simulink model "receiver"  (R2021b)
settings: Solver=VariableStepAuto  StartTime=0.0  StopTime=10000/3.2e6  RelTol=1e-3
PreLoadFcn:
  | setup_receiver
InitFcn:
  | setup_receiver
values from neighbouring files (symbols this model uses):
  fir_bbuf = reshape([fir_barker_13; fir_barker_13; fir_barker_13], [1, length(fir_barker_13)*3])    [setup_receiver.m]
  tx_data = [tx_data mbuf]    [setup_receiver.m]
undefined symbols (not defined in the file or in its folder): AXI4, designMultirateFIR, Lite, xlfda_numerator
libraries: hdlBasic x467, hdlsllib x15, dspmlti4 x8, hdlDSPIP x6, hdlSSR x6, dspswit3 x4, hdlUtilities x3, commrandsrc3 x2, dspsigops x2, simulink x1, vmcUtilities x1
(part 2 of 6)

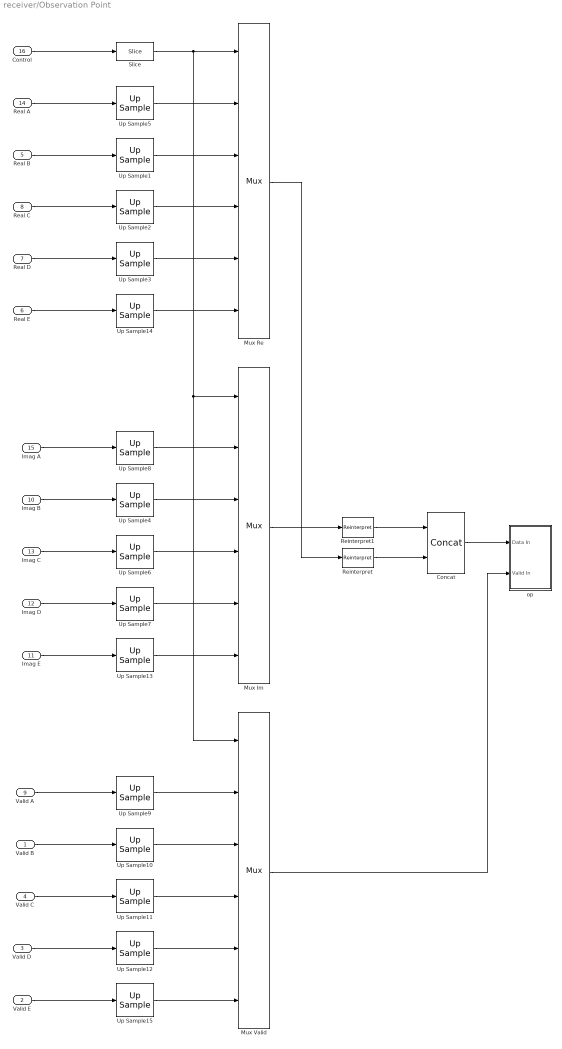
== system receiver/Observation Point ==
  Valid B : Inport
  Valid E : Inport  Port=2
  Valid D : Inport  Port=3
  Valid C : Inport  Port=4
  Real B : Inport  Port=5
  Real E : Inport  Port=6
  Real D : Inport  Port=7
  Real C : Inport  Port=8
  Valid A : Inport  Port=9
  Imag B : Inport  Port=10
  Imag E : Inport  Port=11
  Imag D : Inport  Port=12
  Imag C : Inport  Port=13
  Real A : Inport  Port=14
  Imag A : Inport  Port=15
  Control : Inport  Port=16
  Concat : hdlBasic/Concat  num_inputs=2  XmcBlockStatus=1  maskContainerNames=group1  block_type=concat  block_config=sysgen:Concat_config
  Mux Im : hdlBasic/Mux  inputs=5  en=off  latency=1  precision=Full  arith_type=Unsigned  n_bits=16  bin_pt=14  quantization=Truncate  overflow=Wrap  XmcBlockStatus=1  maskContainerNames=tabcontainer1  block_type=mux  block_config=sysgen:Mux_config
  Mux Re : hdlBasic/Mux  inputs=5  en=off  latency=1  precision=Full  arith_type=Unsigned  n_bits=16  bin_pt=14  quantization=Truncate  overflow=Wrap  XmcBlockStatus=1  maskContainerNames=tabcontainer1  block_type=mux  block_config=sysgen:Mux_config
  Mux Valid : hdlBasic/Mux  inputs=5  en=off  latency=1  precision=Full  arith_type=Unsigned  n_bits=16  bin_pt=14  quantization=Truncate  overflow=Wrap  XmcBlockStatus=1  maskContainerNames=tabcontainer1  block_type=mux  block_config=sysgen:Mux_config
  Reinterpret : hdlBasic/Reinterpret  force_arith_type=on  arith_type=Unsigned  force_bin_pt=on  bin_pt=0  XmcBlockStatus=1  maskContainerNames=group1  block_type=reinterpret  block_config=sysgen:Reinterpret_config
  Reinterpret1 : hdlBasic/Reinterpret  force_arith_type=on  arith_type=Unsigned  force_bin_pt=on  bin_pt=0  XmcBlockStatus=1  maskContainerNames=group1  block_type=reinterpret  block_config=sysgen:Reinterpret_config
  Slice : hdlBasic/Slice  nbits=1  boolean_output=off  mode=Two Bit Locations  bit1=2  base1=LSB of Input  bit0=0  base0=LSB of Input  XmcBlockStatus=1  maskContainerNames=group1  block_type=slice  block_config=sysgen:Slice_config
  Up Sample{1..2,4..6,8} (6 alike) : hdlBasic/Up Sample  sample_ratio=64e6/3.2e6  copy_samples=on  en=off  latency=0  XmcBlockStatus=1  maskContainerNames=group1  block_type=usamp  block_config=sysgen:Upsample_config
  Up Sample10 : hdlBasic/Up Sample  sample_ratio=64e6/3.2e6  copy_samples=off  en=off  latency=0  XmcBlockStatus=1  maskContainerNames=group1  block_type=usamp  block_config=sysgen:Upsample_config
  Up Sample11 : hdlBasic/Up Sample  sample_ratio=64e6/3.2e6  copy_samples=off  en=off  latency=0  XmcBlockStatus=1  maskContainerNames=group1  block_type=usamp  block_config=sysgen:Upsample_config
  Up Sample12 : hdlBasic/Up Sample  sample_ratio=64e6/12.8e6  copy_samples=off  en=off  latency=0  XmcBlockStatus=1  maskContainerNames=group1  block_type=usamp  block_config=sysgen:Upsample_config
  Up Sample{3,7,13..14} (4 alike) : hdlBasic/Up Sample  sample_ratio=64e6/12.8e6  copy_samples=on  en=off  latency=0  XmcBlockStatus=1  maskContainerNames=group1  block_type=usamp  block_config=sysgen:Upsample_config
  Up Sample15 : hdlBasic/Up Sample  sample_ratio=64e6/12.8e6  copy_samples=off  en=off  latency=0  XmcBlockStatus=1  maskContainerNames=group1  block_type=usamp  block_config=sysgen:Upsample_config
  Up Sample9 : hdlBasic/Up Sample  sample_ratio=64e6/3.2e6  copy_samples=off  en=off  latency=0  XmcBlockStatus=1  maskContainerNames=group1  block_type=usamp  block_config=sysgen:Upsample_config
  op : Subsystem
  wires:
  Valid B/1 -> Up Sample10/1
  Up Sample10/1 -> Mux Valid/3
  Control/1 -> Slice/1
  Up Sample1/1 -> Mux Re/3
  Concat/1 -> op/1(Data In)
  Mux Re/1 -> Reinterpret/1
  Real B/1 -> Up Sample1/1
  Up Sample11/1 -> Mux Valid/4
  Up Sample2/1 -> Mux Re/4
  Mux Valid/1 -> op/2(Valid In)
  Up Sample3/1 -> Mux Re/5
  Up Sample6/1 -> Mux Im/4
  Up Sample12/1 -> Mux Valid/5
  Imag A/1 -> Up Sample8/1
  Real A/1 -> Up Sample5/1
  Reinterpret/1 -> Concat/2
  Up Sample7/1 -> Mux Im/5
  Reinterpret1/1 -> Concat/1
  Imag C/1 -> Up Sample6/1
  Up Sample5/1 -> Mux Re/2
  Up Sample4/1 -> Mux Im/3
  Up Sample8/1 -> Mux Im/2
  Mux Im/1 -> Reinterpret1/1
  Up Sample9/1 -> Mux Valid/2
  Valid A/1 -> Up Sample9/1
  Imag D/1 -> Up Sample7/1
  Valid D/1 -> Up Sample12/1
  Real D/1 -> Up Sample3/1
  Valid C/1 -> Up Sample11/1
  Valid E/1 -> Up Sample15/1
  Imag E/1 -> Up Sample13/1
  Real C/1 -> Up Sample2/1
  Imag B/1 -> Up Sample4/1
  Real E/1 -> Up Sample14/1
  Slice/1 -> Mux Valid/1, Mux Im/1, Mux Re/1
  Up Sample13/1 -> Mux Im/6
  Up Sample14/1 -> Mux Re/6
  Up Sample15/1 -> Mux Valid/6

== system receiver/QPSK System ==
  Enable : Inport
  Complex to Real-Imag : ComplexToRealImag
  QPSK TX Generation : Subsystem
  RF Balun Gain RX : Gain  Gain=1/2
  RF Balun Gain TX : Gain  Gain=1/2
  RF-ADC : Subsystem  mask{fs_ghz=1.024, decim=8x, ssr=2, mode=Fine, fc=0.064100, fph=0, fcoarse=fs/4}
      mask prompts: fs_ghz "Sample Rate (GHz):"; decim "Interpolation Mode:"; ssr "Samples per AXI4-Stream Cycle:"; mode "Mixer Type:"; fc "NCO Frequency (GHz):"; fph "NCO Phase (Rads):"; fcoarse "Frequency:"
      mask init:
      | % Obtain the sample rate in Hz
      | fs = str2double(get_param(gcb, 'fs_ghz'))*1e9;
      | 
      | % Set the mode of the RF-DAC interpolation filter
      | switch get_param(gcb, 'decim')
      |     case '1x'
      |         D = 1;
      |     case '2x'
      |         D = 2;
      |     case '4x'
      |         D = 4;
      |     case '8x'
      |         D = 8;
      |     otherwise
      |         D = 1;
      | end
      | 
      | % Get the AXI-Stream clock for display to user
      | axi_clk = (fs/(str2double(get_param(gcb, 'ssr'))*D))*1e-6;
      | 
      | % Get the block mask object to manipulate settings
      | mo = get_param(gcb, 'MaskObject');
      | 
      | % Update text to display the required AXI-Stream clock
      | tc = mo.getDialogControl('axi_text');
      | tc.Prompt = ['      Required AXI-Stream Clock: ', num2str(axi_clk), ' MHz'];
      | 
      | % Set the RF-DAC Mixer mode
      | switch get_param(gcb, 'mode')
      |     case 'Bypass'
      |         m = 0;
      |     case 'Coarse'
      |         m = 1;
      |     case 'Fine'
      |         m = 2;
      |     otherwise
      |         m = 0;
      | end
      | 
      | % Set the RF-DAC Coarse Mixer mode
      | switch get_param(gcb, 'fcoarse')
      |     case 'fs/2'
      |         mc = 0;
      |     case 'fs/4'
      |         mc = 1;
      |     case '-fs/4'
      |         mc = 2;
      |     otherwise
      |         mc = 0;
      | end
      | 
      | % Set other blocks
      | set_param([gcb, '/Decimation Filter'], 'decim', get_param(gcb, 'decim'));
      mask Callback fs_ghz:
      | % Obtain the sample rate in Hz
      | fs = str2double(get_param(gcb, 'fs_ghz'))*1e9;
      | 
      | % Set the mode of the RF-DAC interpolation filter
      | switch get_param(gcb, 'decim')
      |     case '1x'
      |         D = 1;
      |     case '2x'
      |         D = 2;
      |     case '4x'
      |         D = 4;
      |     case '8x'
      |         D = 8;
      |     otherwise
      |         D = 1;
      | end
      | 
      | % Get the AXI-Stream clock for display to user
      | axi_clk = (fs/(str2double(get_param(gcb, 'ssr'))*D))*1e-6;
      | 
      | % Get the block mask object to manipulate settings
      | mo = get_param(gcb, 'MaskObject');
      | 
      | % Update text to display the required AXI-Stream clock
      | tc = mo.getDialogControl('axi_text');
      | tc.Prompt = ['      Required AXI-Stream Clock: ', num2str(axi_clk), ' MHz'];
      mask TypeOptions decim: 1x | 2x | 4x | 8x
      mask Callback decim:
      | % Obtain the sample rate in Hz
      | fs = str2double(get_param(gcb, 'fs_ghz'))*1e9;
      | 
      | % Set the mode of the RF-DAC interpolation filter
      | switch get_param(gcb, 'decim')
      |     case '1x'
      |         D = 1;
      |     case '2x'
      |         D = 2;
      |     case '4x'
      |         D = 4;
      |     case '8x'
      |         D = 8;
      |     otherwise
      |         D = 1;
      | end
      | 
      | % Get the AXI-Stream clock for display to user
      | axi_clk = (fs/(str2double(get_param(gcb, 'ssr'))*D))*1e-6;
      | 
      | % Get the block mask object to manipulate settings
      | mo = get_param(gcb, 'MaskObject');
      | 
      | % Update text to display the required AXI-Stream clock
      | tc = mo.getDialogControl('axi_text');
      | tc.Prompt = ['      Required AXI-Stream Clock: ', num2str(axi_clk), ' MHz'];
      mask TypeOptions ssr: 1 | 2 | 3 | 4 | 5 | 6 | 7 | 8 | 9 | 10 | 11 | 12 | 13 | 14 | 15 | 16
      mask Callback ssr:
      | % Obtain the sample rate in Hz
      | fs = str2double(get_param(gcb, 'fs_ghz'))*1e9;
      | 
      | % Set the mode of the RF-DAC interpolation filter
      | switch get_param(gcb, 'decim')
      |     case '1x'
      |         D = 1;
      |     case '2x'
      |         D = 2;
      |     case '4x'
      |         D = 4;
      |     case '8x'
      |         D = 8;
      |     otherwise
      |         D = 1;
      | end
      | 
      | % Get the AXI-Stream clock for display to user
      | axi_clk = (fs/(str2double(get_param(gcb, 'ssr'))*D))*1e-6;
      | 
      | % Get the block mask object to manipulate settings
      | mo = get_param(gcb, 'MaskObject');
      | 
      | % Update text to display the required AXI-Stream clock
      | tc = mo.getDialogControl('axi_text');
      | tc.Prompt = ['      Required AXI-Stream Clock: ', num2str(axi_clk), ' MHz'];
      mask TypeOptions mode: Coarse | Fine
      mask Callback mode:
      | % Get the block mask object to manipulate settings
      | mo = get_param(gcb, 'MaskObject');
      | 
      | % Hide group depending on Mixer mode choice
      | switch get_param(gcb, 'mode')
      |     case 'Bypass'
      |         mo.getDialogControl('coarse_group').Visible='off';
      |         mo.getDialogControl('mixer_group').Visible='off';
      |     case 'Coarse'
      |         mo.getDialogControl('coarse_group').Visible='on';
      |         mo.getDialogControl('mixer_group').Visible='off';
      |     case 'Fine'
      |         mo.getDialogControl('coarse_group').Visible='off';
      |         mo.getDialogControl('mixer_group').Visible='on';
      |     otherwise
      |         mo.getDialogControl('coarse_group').Visible='off';
      |         mo.getDialogControl('mixer_group').Visible='off';
      | end
      mask TypeOptions fcoarse: fs/2 | fs/4 | -fs/4
      mask DialogControl DescGroupVar Prompt: RF-DAC
      mask DialogControl DescTextVar Prompt: This block simulates one RF-ADC channel.
      mask DialogControl main_group Prompt: Data Settings
      mask DialogControl axi_text Prompt: Required AXI-Stream Clock: 64 MHz
      mask DialogControl Container5 Prompt: Mixer Settings
  RF-DAC : Subsystem  mask{fs_ghz=1.024, interp=8x, ssr=1, mode=Fine, fc=0.064, fph=0, fcoarse=fs/4}
      mask prompts: fs_ghz "Sample Rate (GHz):"; interp "Interpolation Mode:"; ssr "Samples per AXI4-Stream Cycle:"; mode "Mixer Type:"; fc "NCO Frequency (GHz):"; fph "NCO Phase (Rads):"; fcoarse "Frequency:"
      mask init:
      | % Obtain the sample rate in Hz
      | fs = str2double(get_param(gcb, 'fs_ghz'))*1e9;
      | 
      | % Set the mode of the RF-DAC interpolation filter
      | switch get_param(gcb, 'interp')
      |     case '1x'
      |         L = 1;
      |     case '2x'
      |         L = 2;
      |     case '4x'
      |         L = 4;
      |     case '8x'
      |         L = 8;
      |     otherwise
      |         L = 1;
      | end
      | 
      | % Get the AXI-Stream clock for display to user
      | axi_clk = (fs/(str2double(get_param(gcb, 'ssr'))*L))*1e-6;
      | 
      | % Get the block mask object to manipulate settings
      | mo = get_param(gcb, 'MaskObject');
      | 
      | % Update text to display the required AXI-Stream clock
      | tc = mo.getDialogControl('axi_text');
      | tc.Prompt = ['      Required AXI-Stream Clock: ', num2str(axi_clk), ' MHz'];
      | 
      | % Set the RF-DAC Mixer mode
      | switch get_param(gcb, 'mode')
      |     case 'Bypass'
      |         m = 0;
      |     case 'Coarse'
      |         m = 1;
      |     case 'Fine'
      |         m = 2;
      |     otherwise
      |         m = 0;
      | end
      | 
      | % Set the RF-DAC Coarse Mixer mode
      | switch get_param(gcb, 'fcoarse')
      |     case 'fs/2'
      |         mc = 0;
      |     case 'fs/4'
      |         mc = 1;
      |     case '-fs/4'
      |         mc = 2;
      |     otherwise
      |         mc = 0;
      | end
      | 
      | % Set other blocks
      | set_param([gcb, '/Interpolation Filter'], 'interp', get_param(gcb, 'interp'));
      mask Callback fs_ghz:
      | % Obtain the sample rate in Hz
      | fs = str2double(get_param(gcb, 'fs_ghz'))*1e9;
      | 
      | % Set the mode of the RF-DAC interpolation filter
      | switch get_param(gcb, 'interp')
      |     case '1x'
      |         L = 1;
      |     case '2x'
      |         L = 2;
      |     case '4x'
      |         L = 4;
      |     case '8x'
      |         L = 8;
      |     otherwise
      |         L = 1;
      | end
      | 
      | % Get the AXI-Stream clock for display to user
      | axi_clk = (fs/(str2double(get_param(gcb, 'ssr'))*L))*1e-6;
      | 
      | % Get the block mask object to manipulate settings
      | mo = get_param(gcb, 'MaskObject');
      | 
      | % Update text to display the required AXI-Stream clock
      | tc = mo.getDialogControl('axi_text');
      | tc.Prompt = ['      Required AXI-Stream Clock: ', num2str(axi_clk), ' MHz'];
      mask TypeOptions interp: 1x | 2x | 4x | 8x
      mask Callback interp:
      | % Obtain the sample rate in Hz
      | fs = str2double(get_param(gcb, 'fs_ghz'))*1e9;
      | 
      | % Set the mode of the RF-DAC interpolation filter
      | switch get_param(gcb, 'interp')
      |     case '1x'
      |         L = 1;
      |     case '2x'
      |         L = 2;
      |     case '4x'
      |         L = 4;
      |     case '8x'
      |         L = 8;
      |     otherwise
      |         L = 1;
      | end
      | 
      | % Get the AXI-Stream clock for display to user
      | axi_clk = (fs/(str2double(get_param(gcb, 'ssr'))*L))*1e-6;
      | 
      | % Get the block mask object to manipulate settings
      | mo = get_param(gcb, 'MaskObject');
      | 
      | % Update text to display the required AXI-Stream clock
      | tc = mo.getDialogControl('axi_text');
      | tc.Prompt = ['      Required AXI-Stream Clock: ', num2str(axi_clk), ' MHz'];
      mask TypeOptions ssr: 1 | 2 | 3 | 4 | 5 | 6 | 7 | 8 | 9 | 10 | 11 | 12 | 13 | 14 | 15 | 16
      mask Callback ssr:
      | % Obtain the sample rate in Hz
      | fs = str2double(get_param(gcb, 'fs_ghz'))*1e9;
      | 
      | % Set the mode of the RF-DAC interpolation filter
      | switch get_param(gcb, 'interp')
      |     case '1x'
      |         L = 1;
      |     case '2x'
      |         L = 2;
      |     case '4x'
      |         L = 4;
      |     case '8x'
      |         L = 8;
      |     otherwise
      |         L = 1;
      | end
      | 
      | % Get the AXI-Stream clock for display to user
      | axi_clk = (fs/(str2double(get_param(gcb, 'ssr'))*L))*1e-6;
      | 
      | % Get the block mask object to manipulate settings
      | mo = get_param(gcb, 'MaskObject');
      | 
      | % Update text to display the required AXI-Stream clock
      | tc = mo.getDialogControl('axi_text');
      | tc.Prompt = ['      Required AXI-Stream Clock: ', num2str(axi_clk), ' MHz'];
      mask TypeOptions mode: Coarse | Fine
      mask Callback mode:
      | % Get the block mask object to manipulate settings
      | mo = get_param(gcb, 'MaskObject');
      | 
      | % Hide group depending on Mixer mode choice
      | switch get_param(gcb, 'mode')
      |     case 'Bypass'
      |         mo.getDialogControl('coarse_group').Visible='off';
      |         mo.getDialogControl('mixer_group').Visible='off';
      |     case 'Coarse'
      |         mo.getDialogControl('coarse_group').Visible='on';
      |         mo.getDialogControl('mixer_group').Visible='off';
      |     case 'Fine'
      |         mo.getDialogControl('coarse_group').Visible='off';
      |         mo.getDialogControl('mixer_group').Visible='on';
      |     otherwise
      |         mo.getDialogControl('coarse_group').Visible='off';
      |         mo.getDialogControl('mixer_group').Visible='off';
      | end
      mask TypeOptions fcoarse: fs/2 | fs/4 | -fs/4
      mask DialogControl DescGroupVar Prompt: RF-DAC
      mask DialogControl DescTextVar Prompt: This block simulates one RF-DAC channel.
      mask DialogControl main_group Prompt: Data Settings
      mask DialogControl axi_text Prompt: Required AXI-Stream Clock: 128 MHz
      mask DialogControl Container5 Prompt: Mixer Settings
  Re : Outport  VectorParamsAs1DForOutWhenUnconnected=off
  Im : Outport  Port=2  VectorParamsAs1DForOutWhenUnconnected=off
  wires:
  QPSK TX Generation/1(QPSK) -> RF-DAC/1(Data In)
  Enable/1 -> QPSK TX Generation/1(Enable)
  Complex to Real-Imag/1 -> Re/1
  Complex to Real-Imag/2 -> Im/1
  RF-ADC/1(Data Out) -> Complex to Real-Imag/1
  RF-DAC/1(Data Out) -> RF Balun Gain TX/1
  RF Balun Gain TX/1 -> RF Balun Gain RX/1
  RF Balun Gain RX/1 -> RF-ADC/1(Data In)

== system receiver/RRC Receive Filter ==
  Valid In : Inport
  Real In : Inport  Port=2
  Imag In : Inport  Port=3
  Convert : hdlBasic/Convert  gui_display_data_type=Fixed-point  arith_type=Signed (2's comp)  n_bits=16  bin_pt=14  float_type=Single  exp_bits=8  fraction_bits=24  quantization=Truncate  overflow=Wrap  en=off  latency=0  pipeline=off  XmcBlockStatus=1  maskContainerNames=group2  block_type=convert  block_config=sysgen:Convert_config  block_width=595  block_height=885
  Convert1 : hdlBasic/Convert  gui_display_data_type=Fixed-point  arith_type=Signed (2's comp)  n_bits=16  bin_pt=14  float_type=Single  exp_bits=8  fraction_bits=24  quantization=Truncate  overflow=Wrap  en=off  latency=0  pipeline=off  XmcBlockStatus=1  maskContainerNames=group2  block_type=convert  block_config=sysgen:Convert_config  block_width=595  block_height=885
  FDATool : hdlUtilities/FDATool  block_type=fdatool
      settings: infoedit=FDATool
  "FIR Compiler 7.2 " : hdlDSPIP/FIR Compiler 7.2   coefficientvector=xlfda_numerator('FDATool')  coefficient_sets=1  coefficient_reload=off  filter_type=Decimation  rate_change_type=Integer  interpolation_rate=1  decimation_rate=4  zero_pack_factor=1  channel_sequence=Basic  number_channels=1  pattern_list='P4-0,P4-1,P4-2,P4-3,P4-4'  number_paths=2  ratespecification=Maximum_Possible  sampleperiod=0.25000000  hardwareoversamplingrate=1  coefficient_sign=Signed  quantization=Quantize_Only  coefficient_width=16  bestprecision=on  coefficient_fractional_bits=16  coefficient_structure=Inferred  output_rounding_mode=Full_Precision  output_width=33  filter_architecture=Systolic_Multiply_Accumulate  optimization_goal=Area  optimization_list='None'  data_buffer_type=Automatic  coefficient_buffer_type=Automatic  input_buffer_type=Automatic  output_buffer_type=Automatic  preference_for_other_storage=Automatic  multi_column_support=Automatic  columnconfig='6'  inter_column_pipe_length=4  data_has_tlast=Not_Required  m_data_has_tready=off  s_data_has_fifo=off  s_data_has_tuser=Not_Required  m_data_has_tuser=Not_Required  s_config_sync_mode=On_Vector  s_config_method=Single  num_reload_slots=1  has_aclken=off  has_aresetn=off  reset_data_vector=on  trim_axipin_name=on  simulation_type=hybrid_sim  simulation_model=sysgen:xfirv7_2_cmodel  data_path_portlist={ 's_axis_data_tdata', 'm_axis_data_tdata' }  passband_min=0.0  passband_max=0.5  stopband_min=0.5  stopband_max=1.0  filter_selection=1  gui_behaviour='Sysgen_GUI'  data_sign=Signed  data_width=16  data_fractional_bits=0  data_tuser_width=1  wrapper_available=true  ip_wrap_arbitrary_binary_point=true  ip_name=FIR Compiler  ip_version=7.2  dsptool_ready=true  ipcore_usecache=true  ipcore_useipmodelcache=true  port_translation_map={ 'aclken' => 'en', 'aresetn' => 'rst' }  run_core_at_system_period=true  ipcore_xco_need_fpga_part=true  ipcore_fpga_part=[]  XmcBlockStatus=1  maskContainerNames=tabcontainer1  block_type=fir_compiler_v7_2  block_config=sysgen:rodinimport_config  block_width=820  block_height=600
  Terminator2 : Terminator
  Terminator4 : Terminator
  Valid Out : Outport  VectorParamsAs1DForOutWhenUnconnected=off
  Real Out : Outport  Port=2  VectorParamsAs1DForOutWhenUnconnected=off
  Imag Out : Outport  Port=3  VectorParamsAs1DForOutWhenUnconnected=off
  wires:
  "FIR Compiler 7.2 "/2 -> Valid Out/1
  "FIR Compiler 7.2 "/4 -> Convert1/1
  Imag In/1 -> "FIR Compiler 7.2 "/2
  "FIR Compiler 7.2 "/1 -> Terminator2/1
  Real In/1 -> "FIR Compiler 7.2 "/1
  Convert/1 -> Real Out/1
  "FIR Compiler 7.2 "/3 -> Convert/1
  Convert1/1 -> Imag Out/1
  Valid In/1 -> Terminator4/1

== system receiver/Reset Subsystem ==
  Global Reset : Inport
  Time Reset In : Inport  Port=2
  Phase Reset In : Inport  Port=3
  Frame Reset In : Inport  Port=4
  Modulation : Inport  Port=5
  Logical{,1..2,4} (4 alike) : hdlBasic/Logical  logical_function=OR  inputs=2  en=off  latency=0  precision=Full  arith_type=Unsigned  n_bits=16  bin_pt=0  align_bp=on  overflow=[]  quantization=[]  XmcBlockStatus=1  maskContainerNames=tabcontainer1  block_type=logical  block_config=sysgen:Logical_config
  Logical3 : hdlBasic/Logical  logical_function=XOR  inputs=2  en=off  latency=0  precision=Full  arith_type=Unsigned  n_bits=16  bin_pt=0  align_bp=on  overflow=[]  quantization=[]  XmcBlockStatus=1  maskContainerNames=tabcontainer1  block_type=logical  block_config=sysgen:Logical_config
  Register : hdlBasic/Register  init=0  rst=off  en=off  XmcBlockStatus=1  maskContainerNames=tabcontainer1  block_type=register  block_config=sysgen:Register_config
  Time Reset Out : Outport
  Phase Reset Out : Outport  Port=2
  Frame Reset Out : Outport  Port=3
  wires:
  Time Reset In/1 -> Logical/2
  Logical/1 -> Time Reset Out/1
  Phase Reset In/1 -> Logical1/2
  Frame Reset In/1 -> Logical2/2
  Logical2/1 -> Frame Reset Out/1
  Logical1/1 -> Phase Reset Out/1
  Modulation/1 -> Logical3/1, Register/1
  Global Reset/1 -> Logical4/1
  Logical4/1 -> Logical2/1, Logical1/1, Logical/1
  Register/1 -> Logical3/2
  Logical3/1 -> Logical4/2

== system receiver/SSR Halfband Lowpass Decimator ==
  Valid In : Inport
  Real In : Inport  Port=2
  Imag In : Inport  Port=3
  Convert : hdlBasic/Convert  gui_display_data_type=Fixed-point  arith_type=Signed (2's comp)  n_bits=16  bin_pt=14  float_type=Single  exp_bits=8  fraction_bits=24  quantization="Round  (unbiased: +/- Inf)"  overflow=Saturate  en=off  latency=0  pipeline=off  XmcBlockStatus=1  maskContainerNames=group2  block_type=convert  block_config=sysgen:Convert_config  block_width=595  block_height=885
  Convert1 : hdlBasic/Convert  gui_display_data_type=Fixed-point  arith_type=Signed (2's comp)  n_bits=16  bin_pt=14  float_type=Single  exp_bits=8  fraction_bits=24  quantization="Round  (unbiased: +/- Inf)"  overflow=Saturate  en=off  latency=0  pipeline=off  XmcBlockStatus=1  maskContainerNames=group2  block_type=convert  block_config=sysgen:Convert_config  block_width=595  block_height=885
  FDATool : hdlUtilities/FDATool  block_type=fdatool
      settings: infoedit=FDATool
  Terminator1 : Terminator
  Terminator2 : Terminator
  Vector FIR Im : hdlSSR/Vector FIR  coefficientvector=xlfda_numerator('FDATool')/(max(xlfda_numerator('FDATool'))*2)  coefficient_sets=1  coefficient_reload=off  filter_type=Decimation  rate_change_type=Integer  interpolation_rate=1  decimation_rate=2  zero_pack_factor=1  sg_ssr=2  coefficient_sign=Signed  quantization=Quantize_Only  coefficient_width=16  bestprecision=off  coefficient_fractional_bits=14  coefficient_structure=Inferred  output_rounding_mode=Full_Precision  output_width=24  filter_architecture=Systolic_Multiply_Accumulate  optimization_goal=Area  optimization_list='None'  data_buffer_type=Automatic  coefficient_buffer_type=Automatic  input_buffer_type=Automatic  output_buffer_type=Automatic  preference_for_other_storage=Automatic  multi_column_support=Automatic  columnconfig='11'  inter_column_pipe_length=4  m_data_has_tready=off  has_aclken=off  has_aresetn=off  reset_data_vector=on  simulation_type=xsim  simulation_model=sysgen:xfirv7_2_cmodel  data_path_portlist={ 's_axis_data_tdata', 'm_axis_data_tdata' }  passband_min=0.0  passband_max=0.5  stopband_min=0.5  stopband_max=1.0  filter_selection=1  gui_behaviour=1  data_sign=Signed  data_width=16  data_fractional_bits=0  data_tuser_width='11'  wrapper_available=true  ip_wrap_arbitrary_binary_point=true  ip_name=FIR Compiler  ip_version=7.2  dsptool_ready=true  ipcore_usecache=true  ipcore_useipmodelcache=true  port_translation_map={ 'aclken' => 'en', 'aresetn' => 'rst' }  run_core_at_system_period=true  ipcore_xco_need_fpga_part=true  ipcore_fpga_part=[]  block_type=fir_compiler_v7_2_ssr  decimation_prev=2  interpolation_prev=1  coeffsets_prev=1  filter_prev=Decimation  channel_sequence=Basic  number_channels=1  pattern_list='P4-0,P4-1,P4-2,P4-3,P4-4'  number_paths=1  data_has_tlast=Not_Required  s_data_has_fifo=off  s_data_has_tuser=Not_Required  m_data_has_tuser=Not_Required  s_config_sync_mode=On_Vector  s_config_method=Single  num_reload_slots=1  XmcBlockStatus=1  sg_ssr_prev=2  maskContainerNames=group10  block_width=657
      settings: SourceProductName=Xilinx SSR Blockset  block_version=1.0
  Vector FIR Re : hdlSSR/Vector FIR  coefficientvector=xlfda_numerator('FDATool')/(max(xlfda_numerator('FDATool'))*2)  coefficient_sets=1  coefficient_reload=off  filter_type=Decimation  rate_change_type=Integer  interpolation_rate=1  decimation_rate=2  zero_pack_factor=1  sg_ssr=2  coefficient_sign=Signed  quantization=Quantize_Only  coefficient_width=16  bestprecision=off  coefficient_fractional_bits=14  coefficient_structure=Inferred  output_rounding_mode=Full_Precision  output_width=24  filter_architecture=Systolic_Multiply_Accumulate  optimization_goal=Area  optimization_list='None'  data_buffer_type=Automatic  coefficient_buffer_type=Automatic  input_buffer_type=Automatic  output_buffer_type=Automatic  preference_for_other_storage=Automatic  multi_column_support=Automatic  columnconfig='11'  inter_column_pipe_length=4  m_data_has_tready=off  has_aclken=off  has_aresetn=off  reset_data_vector=on  simulation_type=xsim  simulation_model=sysgen:xfirv7_2_cmodel  data_path_portlist={ 's_axis_data_tdata', 'm_axis_data_tdata' }  passband_min=0.0  passband_max=0.5  stopband_min=0.5  stopband_max=1.0  filter_selection=1  gui_behaviour=1  data_sign=Signed  data_width=16  data_fractional_bits=0  data_tuser_width='11'  wrapper_available=true  ip_wrap_arbitrary_binary_point=true  ip_name=FIR Compiler  ip_version=7.2  dsptool_ready=true  ipcore_usecache=true  ipcore_useipmodelcache=true  port_translation_map={ 'aclken' => 'en', 'aresetn' => 'rst' }  run_core_at_system_period=true  ipcore_xco_need_fpga_part=true  ipcore_fpga_part=[]  block_type=fir_compiler_v7_2_ssr  decimation_prev=2  interpolation_prev=1  coeffsets_prev=1  filter_prev=Decimation  channel_sequence=Basic  number_channels=1  pattern_list='P4-0,P4-1,P4-2,P4-3,P4-4'  number_paths=1  data_has_tlast=Not_Required  s_data_has_fifo=off  s_data_has_tuser=Not_Required  m_data_has_tuser=Not_Required  s_config_sync_mode=On_Vector  s_config_method=Single  num_reload_slots=1  XmcBlockStatus=1  sg_ssr_prev=2  maskContainerNames=group10  block_width=657
      settings: SourceProductName=Xilinx SSR Blockset  block_version=1.0
  Valid Out : Outport  VectorParamsAs1DForOutWhenUnconnected=off
  Real Out : Outport  Port=2  VectorParamsAs1DForOutWhenUnconnected=off
  Imag Out : Outport  Port=3  VectorParamsAs1DForOutWhenUnconnected=off
  Ready Out : Outport  Port=4  VectorParamsAs1DForOutWhenUnconnected=off
  wires:
  Convert1/1 -> Imag Out/1
  Convert/1 -> Real Out/1
  Vector FIR Im/2 -> Terminator2/1
  Vector FIR Re/1 -> Ready Out/1
  Vector FIR Im/1 -> Terminator1/1
  Vector FIR Im/3 -> Convert1/1
  Vector FIR Re/3 -> Convert/1
  Real In/1 -> Vector FIR Re/2
  Vector FIR Re/2 -> Valid Out/1
  Valid In/1 -> Vector FIR Re/1, Vector FIR Im/1
  Imag In/1 -> Vector FIR Im/2

== system receiver/Time Synchronisation ==
  Reset : Inport
  Valid In : Inport  Port=2
  Real In : Inport  Port=3
  Imag In : Inport  Port=4
  Loop Filter : Subsystem  mask{T=1/100e3, d=1/sqrt(2), Kp=1, Bn=100e3*0.05, Ko=1}
      mask prompts: T "Sampling Period:"; d "Damping Ratio:"; Kp "Phase Detector Gain:"; Bn "Noise Bandwidth:"; Ko "Oscillator Gain:"
      mask init:
      | n = (Bn*T)/(d+1/(4*d));
      | 
      | K1 = ((4*d*n)/(1+2*d*n+n^2))/(Ko*Kp);
      | 
      | K2 = ((4*n^2)/(1+2*d*n+n^2))/(Ko*Kp);
      | 
      | %K1 = (4*d*n)/(Ko*Kp);
      | 
      | %K2 = (4*(n^2))/(Ko*Kp);
      mask DialogControl DescGroupVar Prompt: Loop Filter
      mask DialogControl DescTextVar Prompt: A simplified loop filter.
      mask DialogControl ParameterGroupVar Prompt: Main
  NCC : Subsystem  mask{r=32, f=58}
      mask prompts: r "Symbol Oversample Factor:"; f "Fractional Bits:"
      mask init:
      | n = ceil(log2(r))+1;
      mask DialogControl DescGroupVar Prompt: Numerically Controlled Clock (NCC)
      mask DialogControl DescTextVar Prompt: The NCC block contains an accumulator that increments by one each clock cycle. The wordlength of the accumulator is determined by the symbol oversampling factor. Once the maximum value of the accumulator is reached, the accumulation starts again. The error signal can be used to increase or decrease the rate of accumulation. When the accumulator wraps around, a binary high is released from the strobe port.
      mask DialogControl ParameterGroupVar Prompt: Main
  Terminator : Terminator
  Timing Error Detector : Subsystem
  Valid Out : Outport  VectorParamsAs1DForOutWhenUnconnected=off
  Real Out : Outport  Port=2  VectorParamsAs1DForOutWhenUnconnected=off
  Imag Out : Outport  Port=3  VectorParamsAs1DForOutWhenUnconnected=off
  wires:
  Valid In/1 -> Terminator/1
  Real In/1 -> Timing Error Detector/1(Real In), Loop Filter/1(Real In)
  Loop Filter/4(Error Out) -> NCC/1(Error)
  Timing Error Detector/1(Error) -> Loop Filter/3(Signal In)
  Imag In/1 -> Loop Filter/2(Imag In), Timing Error Detector/2(Imag In)
  Loop Filter/3(Valid Out) -> Valid Out/1
  Loop Filter/1(Real Out) -> Real Out/1
  Loop Filter/2(Imag Out) -> Imag Out/1
  NCC/1(Strobe) -> Loop Filter/4(Valid In)
  Reset/1 -> Loop Filter/5(Reset)

== system receiver/AXI-Stream Master Interface/Rising Edge Detector Enable ==
  Input : Inport
  Inverter2 : hdlBasic/Inverter  en=off  latency=0  XmcBlockStatus=1  maskContainerNames=group2  block_type=inv  block_config=sysgen:Inverter_config
  Logical3 : hdlBasic/Logical  logical_function=AND  inputs=2  en=off  latency=0  precision=Full  arith_type=Unsigned  n_bits=16  bin_pt=0  align_bp=on  overflow=[]  quantization=[]  XmcBlockStatus=1  maskContainerNames=tabcontainer1  block_type=logical  block_config=sysgen:Logical_config
  Register1 : hdlBasic/Register  init=0  rst=off  en=off  XmcBlockStatus=1  maskContainerNames=tabcontainer1  block_type=register  block_config=sysgen:Register_config
  Output : Outport  VectorParamsAs1DForOutWhenUnconnected=off
  wires:
  Input/1 -> Logical3/2, Inverter2/1
  Inverter2/1 -> Register1/1
  Logical3/1 -> Output/1
  Register1/1 -> Logical3/1

== system receiver/AXI-Stream Master Interface/Rising Edge Detector Last ==
  Input : Inport
  Inverter2 : hdlBasic/Inverter  en=off  latency=0  XmcBlockStatus=1  maskContainerNames=group2  block_type=inv  block_config=sysgen:Inverter_config
  Logical3 : hdlBasic/Logical  logical_function=AND  inputs=2  en=off  latency=0  precision=Full  arith_type=Unsigned  n_bits=16  bin_pt=0  align_bp=on  overflow=[]  quantization=[]  XmcBlockStatus=1  maskContainerNames=tabcontainer1  block_type=logical  block_config=sysgen:Logical_config
  Register1 : hdlBasic/Register  init=0  rst=off  en=off  XmcBlockStatus=1  maskContainerNames=tabcontainer1  block_type=register  block_config=sysgen:Register_config
  Output : Outport  VectorParamsAs1DForOutWhenUnconnected=off
  wires:
  Register1/1 -> Logical3/1
  Logical3/1 -> Output/1
  Inverter2/1 -> Register1/1
  Input/1 -> Inverter2/1, Logical3/2

== system receiver/Carrier Synchronisation/De-Rotate Constellation ==
  Imag In : Inport
  Real In : Inport  Port=2
  Valid In : Inport  Port=3
  Imag Error : Inport  Port=4
  Real Error : Inport  Port=5
  Valid Error : Inport  Port=6
  Delay : hdlBasic/Delay  rst=off  en=off  latency=4  reg_retiming=off  XmcBlockStatus=1  maskContainerNames=group1  block_type=delay  block_config=sysgen:Delay_config
  Product : hdlBasic/Product  complex_multiplier=on  optimizegoal=Performance  simulation_type=fast_sim  simulation_model=sysgen:product_macro  XmcBlockStatus=1  maskContainerNames=<empty>  block_type=product_macro  block_config=sysgen:ProductMacro_config
  Register{,1..3} (4 alike) : hdlBasic/Register  init=0  rst=off  en=on  XmcBlockStatus=1  maskContainerNames=tabcontainer1  block_type=register  block_config=sysgen:Register_config
  Register{4..7} (4 alike) : hdlBasic/Register  init=0  rst=off  en=off  XmcBlockStatus=1  maskContainerNames=tabcontainer1  block_type=register  block_config=sysgen:Register_config
  Imag Out : Outport  VectorParamsAs1DForOutWhenUnconnected=off
  Real Out : Outport  Port=2  VectorParamsAs1DForOutWhenUnconnected=off
  Valid Out : Outport  Port=3  VectorParamsAs1DForOutWhenUnconnected=off
  wires:
  Product/2 -> Register1/1
  Product/1 -> Register/1
  Register3/1 -> Product/4
  Register2/1 -> Product/3
  Register5/1 -> Product/2
  Register6/1 -> Product/1
  Delay/1 -> Register4/1, Register1/2, Register/2
  Valid Error/1 -> Register2/2, Register3/2
  Real In/1 -> Register6/1
  Imag In/1 -> Register5/1
  Real Error/1 -> Register2/1
  Register7/1 -> Delay/1
  Register4/1 -> Valid Out/1
  Imag Error/1 -> Register3/1
  Valid In/1 -> Register7/1
  Register1/1 -> Imag Out/1
  Register/1 -> Real Out/1

== system receiver/Carrier Synchronisation/Generate Angle Error ==
  Imag In : Inport
  Real In : Inport  Port=2
  Valid In : Inport  Port=3
  Modulation : Inport  Port=4
  AddSub : hdlBasic/AddSub  mode=Subtraction  use_carryin=off  use_carryout=off  en=off  latency=1  precision=User Defined  arith_type="Signed  (2's comp)"  n_bits=22  bin_pt=20  quantization=Truncate  overflow=Wrap  use_behavioral_HDL=off  hw_selection=Fabric  pipelined=off  XmcBlockStatus=1  maskContainerNames=tabcontainer1  block_type=addsub  block_config=sysgen:Addsub_config
  Circular CORDIC : Subsystem
  Concat : hdlBasic/Concat  num_inputs=2  XmcBlockStatus=1  maskContainerNames=group1  block_type=concat  block_config=sysgen:Concat_config
  Delay : hdlBasic/Delay  rst=off  en=off  latency=11  reg_retiming=off  XmcBlockStatus=1  maskContainerNames=group1  block_type=delay  block_config=sysgen:Delay_config
  Delay1 : hdlBasic/Delay  rst=off  en=off  latency=10  reg_retiming=off  XmcBlockStatus=1  maskContainerNames=group1  block_type=delay  block_config=sysgen:Delay_config
  Im MSB : hdlBasic/Slice  nbits=1  boolean_output=off  mode=Upper Bit Location + Width  bit1=0  base1=MSB of Input  bit0=0  base0=LSB of Input  XmcBlockStatus=1  maskContainerNames=group1  block_type=slice  block_config=sysgen:Slice_config
  Mux : hdlBasic/Mux  inputs=2  en=off  latency=0  precision=Full  arith_type=Unsigned  n_bits=16  bin_pt=14  quantization=Truncate  overflow=Wrap  XmcBlockStatus=1  maskContainerNames=tabcontainer1  block_type=mux  block_config=sysgen:Mux_config
  ROM : hdlBasic/ROM  depth=4  initVector=[pi/4 -pi/4 -pi/4 pi/4]  distributed_mem=Block RAM  rst=off  init_reg=0  en=off  latency=1  gui_display_data_type=Fixed-point  arith_type="Signed  (2's comp)"  n_bits=16  bin_pt=14  preci_type=Single  exp_width=8  frac_width=24  optimize=Area  use_rpm=on  simulation_type=fast_sim  XmcBlockStatus=1  maskContainerNames=tabcontainer1  block_type=sprom  block_config=sysgen:SPROM_config
  Re MSB : hdlBasic/Slice  nbits=1  boolean_output=off  mode=Upper Bit Location + Width  bit1=0  base1=MSB of Input  bit0=0  base0=LSB of Input  XmcBlockStatus=1  maskContainerNames=group1  block_type=slice  block_config=sysgen:Slice_config
  Register : hdlBasic/Register  init=0  rst=off  en=on  XmcBlockStatus=1  maskContainerNames=tabcontainer1  block_type=register  block_config=sysgen:Register_config
  Register1 : hdlBasic/Register  init=0  rst=off  en=on  XmcBlockStatus=1  maskContainerNames=tabcontainer1  block_type=register  block_config=sysgen:Register_config
  Register2 : hdlBasic/Register  init=0  rst=off  en=off  XmcBlockStatus=1  maskContainerNames=tabcontainer1  block_type=register  block_config=sysgen:Register_config
  Register3 : hdlBasic/Register  init=0  rst=off  en=off  XmcBlockStatus=1  maskContainerNames=tabcontainer1  block_type=register  block_config=sysgen:Register_config
  Register4 : hdlBasic/Register  init=0  rst=off  en=off  XmcBlockStatus=1  maskContainerNames=tabcontainer1  block_type=register  block_config=sysgen:Register_config
  Angle : Outport  VectorParamsAs1DForOutWhenUnconnected=off
  Valid Out : Outport  Port=2  VectorParamsAs1DForOutWhenUnconnected=off
  wires:
  Modulation/1 -> Mux/1
  Register4/1 -> Mux/2
  Mux/1 -> Angle/1
  AddSub/1 -> Mux/3
  Register2/1 -> Valid Out/1
  Delay/1 -> Register2/1
  Circular CORDIC/1(Angle) -> Register4/1, AddSub/1
  ROM/1 -> AddSub/2
  Delay1/1 -> ROM/1
  Concat/1 -> Delay1/1
  Im MSB/1 -> Concat/2
  Re MSB/1 -> Concat/1
  Register/1 -> Circular CORDIC/2(Real In), Re MSB/1
  Register3/1 -> Delay/1
  Register1/1 -> Circular CORDIC/1(Imag In), Im MSB/1
  Imag In/1 -> Register1/1
  Real In/1 -> Register/1
  Valid In/1 -> Register1/2, Register/2, Register3/1

== system receiver/Carrier Synchronisation/Generate NCO ==
  Angle : Inport
  Valid In : Inport  Port=2
  Reset : Inport  Port=3
  Loop Filter : Subsystem  mask{T=1/(100e3), d=0.707, Kp=1, Bn=0.001*100e3, Ko=1}
      mask prompts: T "Sampling Period:"; d "Damping Ratio:"; Kp "Phase Detector Gain:"; Bn "Noise Bandwidth:"; Ko "Oscillator Gain:"
      mask init:
      | n = (Bn*T)/(d+1/(4*d));
      | 
      | %K1 = ((4*d*n)/(1+2*d*n+n^2))/(Ko*Kp);
      | 
      | %K2 = ((4*n^2)/(1+2*d*n+n^2))/(Ko*Kp);
      | 
      | K1 = (4*d*n)/(Ko*Kp);
      | 
      | K2 = (4*(n^2))/(Ko*Kp);
  NCO : Subsystem  mask(NCO){n=12, b=36}
      mask prompts: n "Number of integer_bits"; b "Number of fractional bits"
      mask help:
      | Numerically Controller Oscillator.
      |
      | Integrates the phase error and generates cosine and negative sign outputs.
      mask init:
      | k_n = ceil(log2((2^n)/(2*pi)));
      mask DialogControl Container3 Prompt: Accumulator
  Imag Out : Outport  VectorParamsAs1DForOutWhenUnconnected=off
  Real Out : Outport  Port=2  VectorParamsAs1DForOutWhenUnconnected=off
  Valid Out : Outport  Port=3  VectorParamsAs1DForOutWhenUnconnected=off
  wires:
  NCO/3(En_out) -> Valid Out/1
  Angle/1 -> Loop Filter/1(Signal)
  Valid In/1 -> Loop Filter/2(Strobe)
  Loop Filter/1(Error) -> NCO/1(Step Size)
  Loop Filter/2(Valid) -> NCO/2(En_in)
  NCO/2(Neg Sin) -> Imag Out/1
  NCO/1(Cos) -> Real Out/1
  Reset/1 -> Loop Filter/3(Reset)

== system receiver/Coarse Frequency Synchronisation/Apply Frequency Offset Correction ==
  Imag In : Inport
  Real In : Inport  Port=2
  cos : Inport  Port=3
  sin : Inport  Port=4
  Convert : hdlBasic/Convert  gui_display_data_type=Fixed-point  arith_type=Signed (2's comp)  n_bits=16  bin_pt=14  float_type=Single  exp_bits=8  fraction_bits=24  quantization=Truncate  overflow=Saturate  en=off  latency=0  pipeline=off  XmcBlockStatus=1  maskContainerNames=group2  block_type=convert  block_config=sysgen:Convert_config  block_width=595  block_height=885
  Convert1 : hdlBasic/Convert  gui_display_data_type=Fixed-point  arith_type=Signed (2's comp)  n_bits=16  bin_pt=14  float_type=Single  exp_bits=8  fraction_bits=24  quantization=Truncate  overflow=Saturate  en=off  latency=0  pipeline=off  XmcBlockStatus=1  maskContainerNames=group2  block_type=convert  block_config=sysgen:Convert_config  block_width=595  block_height=885
  Product : hdlBasic/Product  complex_multiplier=on  optimizegoal=Performance  simulation_type=fast_sim  simulation_model=sysgen:product_macro  XmcBlockStatus=1  maskContainerNames=<empty>  block_type=product_macro  block_config=sysgen:ProductMacro_config
  Imag Out : Outport  VectorParamsAs1DForOutWhenUnconnected=off
  Real Out : Outport  Port=2  VectorParamsAs1DForOutWhenUnconnected=off
  wires:
  Product/1 -> Convert/1
  Product/2 -> Convert1/1
  Imag In/1 -> Product/2
  Real In/1 -> Product/1
  cos/1 -> Product/3
  sin/1 -> Product/4
  Convert/1 -> Real Out/1
  Convert1/1 -> Imag Out/1

== system receiver/Coarse Frequency Synchronisation/Get Frequency Offset ==
  Mag In : Inport
  SoF : Inport  Port=2
  Constant : hdlBasic/Constant  const=8191  gui_display_data_type=Fixed-point  arith_type=Unsigned  n_bits=13  bin_pt=0  preci_type=Single  exp_width=8  frac_width=24  explicit_period=off  period=1  XmcBlockStatus=1  maskContainerNames=tabcontainer1  block_type=constant  block_config=sysgen:Constant_config
  Counter : hdlBasic/Counter  cnt_type=Count limited  cnt_to=8191  operation=Up  start_count=0  cnt_by_val=1  arith_type=Unsigned  n_bits=13  bin_pt=0  load_pin=off  rst=on  en=off  explicit_period=Inferred from inputs  period=1  use_behavioral_HDL=off  implementation=Fabric  XmcBlockStatus=1  maskContainerNames=group1  block_type=counter  block_config=sysgen:Counter_config  block_width=531  block_height=1023
  ROM : hdlBasic/ROM  depth=8192  initVector=[0:-1:-8192/2+1, 8192/2:-1:1]*(12.8e6/(8192*4))  distributed_mem=Block RAM  rst=off  init_reg=0  en=off  latency=1  gui_display_data_type=Fixed-point  arith_type="Signed  (2's comp)"  n_bits=32  bin_pt=32-ceil(log2(12.8e6/8))-1  preci_type=Single  exp_width=8  frac_width=24  optimize=Area  use_rpm=on  simulation_type=fast_sim  XmcBlockStatus=1  maskContainerNames=tabcontainer1  block_type=sprom  block_config=sysgen:SPROM_config
  Register{,1,5..6} (4 alike) : hdlBasic/Register  init=0  rst=off  en=on  XmcBlockStatus=1  maskContainerNames=tabcontainer1  block_type=register  block_config=sysgen:Register_config
  Register2 : hdlBasic/Register  init=0  rst=off  en=off  XmcBlockStatus=1  maskContainerNames=tabcontainer1  block_type=register  block_config=sysgen:Register_config
  Register3 : hdlBasic/Register  init=0  rst=off  en=off  XmcBlockStatus=1  maskContainerNames=tabcontainer1  block_type=register  block_config=sysgen:Register_config
  Register4 : hdlBasic/Register  init=0  rst=on  en=on  XmcBlockStatus=1  maskContainerNames=tabcontainer1  block_type=register  block_config=sysgen:Register_config
  Relational : hdlBasic/Relational  mode=a=b  op_type=Bool  en=off  latency=0  XmcBlockStatus=1  maskContainerNames=tabcontainer1  block_type=relational  block_config=sysgen:Relational_config
  Relational1 : hdlBasic/Relational  mode=a=b  op_type=Bool  en=off  latency=0  XmcBlockStatus=1  maskContainerNames=tabcontainer1  block_type=relational  block_config=sysgen:Relational_config
  Relational2 : hdlBasic/Relational  mode=a>b  op_type=Bool  en=off  latency=0  XmcBlockStatus=1  maskContainerNames=tabcontainer1  block_type=relational  block_config=sysgen:Relational_config
  Offset Out : Outport  VectorParamsAs1DForOutWhenUnconnected=off
  wires:
  Register6/1 -> ROM/1
  Relational1/1 -> Register6/2
  Register5/1 -> Relational1/2, Register6/1
  Register1/1 -> Register5/1, Relational1/1
  ROM/1 -> Offset Out/1
  Register2/1 -> Register1/2, Register5/2
  Register3/1 -> Register4/1, Relational2/1
  SoF/1 -> Counter/1
  Counter/1 -> Relational/2, Register/1
  Constant/1 -> Relational/1
  Relational/1 -> Register2/1, Register4/2
  Register4/1 -> Relational2/2
  Relational2/1 -> Register/2, Register4/3
  Register/1 -> Register1/1
  Mag In/1 -> Register3/1
